simulink model "WeightedHinfModel"  (R2018b)
settings: Solver=VariableStepAuto  StartTime=0.0  StopTime=10.0  RelTol=1e-3
undefined symbols (not defined in the file): A, B1, B2, C
libraries: cstblocks x4
settings Model: Creator=jban039  LastModifiedBy=jban039

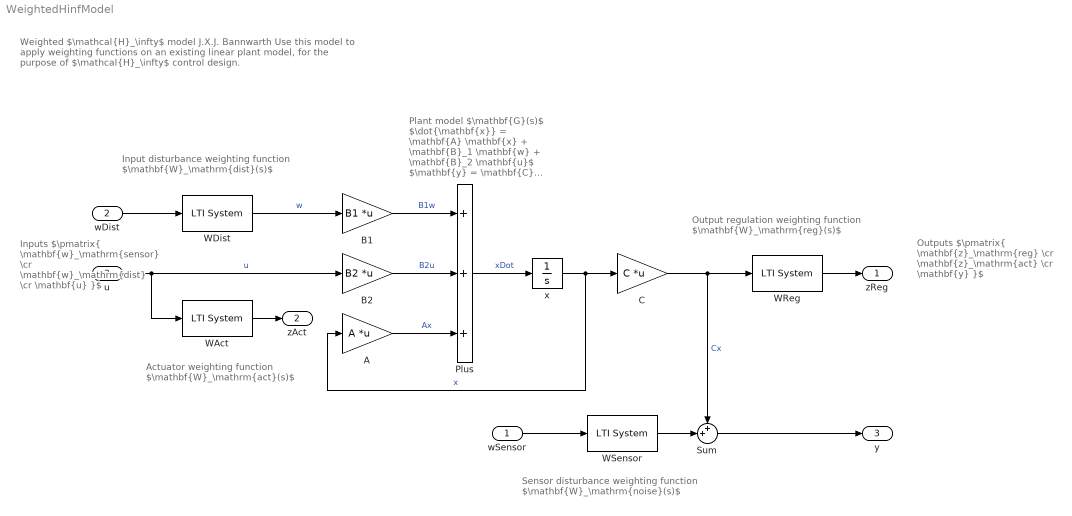
== system WeightedHinfModel ==
  note: Weighted $\mathcal{H}_\infty$ model
      | J.X.J. Bannwarth
      |
      | Use this model to apply weighting functions on an existing
      | linear plant model, for the purpose of $\mathcal{H}_\infty$ control design.
  note: Outputs
      | $\pmatrix{ \mathbf{z}_\mathrm{reg} \cr \mathbf{z}_\mathrm{act} \cr \mathbf{y} }$
  note: Input disturbance weighting function
      | $\mathbf{W}_\mathrm{dist}(s)$
  note: Plant model
      | $\mathbf{G}(s)$
      | $\dot{\mathbf{x}} = \mathbf{A} \mathbf{x} + \mathbf{B}_1 \mathbf{w} + \mathbf{B}_2 \mathbf{u}$
      | $\mathbf{y} = \mathbf{C} \mathbf{x}$
  note: Actuator weighting function
      | $\mathbf{W}_\mathrm{act}(s)$
  note: Sensor disturbance weighting function
      | $\mathbf{W}_\mathrm{noise}(s)$
  note: Output regulation weighting function
      | $\mathbf{W}_\mathrm{reg}(s)$
  note: Inputs
      | $\pmatrix{ \mathbf{w}_\mathrm{sensor} \cr \mathbf{w}_\mathrm{dist} \cr \mathbf{u} }$
  wSensor : Inport
  wDist : Inport  Port=2
  u : Inport  Port=3
  A : Gain  Gain=A  Multiplication=Matrix(K*u)
  B1 : Gain  Gain=B1  Multiplication=Matrix(K*u)
  B2 : Gain  Gain=B2  Multiplication=Matrix(K*u)
  C : Gain  Gain=C  Multiplication=Matrix(K*u)
  Plus : Sum  Inputs=+++
  Sum : Sum  Inputs=++|
  WAct : cstblocks/LTI System  sys=WAct  IC=[]
  WDist : cstblocks/LTI System  sys=WDist  IC=[]
  WReg : cstblocks/LTI System  sys=WReg  IC=[]
  WSensor : cstblocks/LTI System  sys=WSensor  IC=[]
  x : Integrator
  zReg : Outport
  zAct : Outport  Port=2
  y : Outport  Port=3
  wires:
  x/1 -> C/1, A/1  "x"
  A/1 -> Plus/3  "Ax"
  Plus/1 -> x/1  "xDot"
  B1/1 -> Plus/1  "B1w"
  B2/1 -> Plus/2  "B2u"
  WDist/1 -> B1/1  "w"
  u/1 -> WAct/1, B2/1  "u"
  C/1 -> Sum/1, WReg/1  "Cx"
  Sum/1 -> y/1
  WReg/1 -> zReg/1
  WAct/1 -> zAct/1
  WSensor/1 -> Sum/2
  wSensor/1 -> WSensor/1
  wDist/1 -> WDist/1
